simulink model "fuzzy_TCLAB_toolbox"  (R2021a)
settings: Solver=ode45  StartTime=0.0  StopTime=600  RelTol=1e-3  EnableMultiTasking=on
libraries: fuzblock x1
settings Model: Creator=Sergio  LastModifiedBy=Sergio
settings SolverCC: AlgebraicLoopSolver=TrustRegion
settings DataIOCC: LimitDataPoints=on  SaveFormat=Array  SignalLoggingSaveFormat=ModelDataLogs  ReturnWorkspaceOutputs=off
settings OptimizationCC: ExpressionDepthLimit=2147483647  LifeSpan=inf
settings DebuggingCC: UnderspecifiedInitializationDetection=Classic  MergeDetectMultiDrivingBlocksExec=none  SolverPrmCheckMsg=warning  FcnCallInpInsideContextMsg=warning  StateNameClashWarn=warning  SFUnexpectedBacktrackingDiag=warning  SFNoUnconditionalDefaultTransitionDiag=warning  SFExecutionAtInitializationDiag=none  SFMachineParentedDataDiag=warning  ArithmeticOperatorsInVariantConditions=warning
settings HardwareCC: ProdBitPerPointer=32  ProdBitPerSizeT=32  ProdBitPerPtrDiffT=32  ProdLargestAtomicFloat=None  ProdIntDivRoundTo=Undefined  ProdEndianess=Unspecified  ProdWordSize=32  ProdHWDeviceType=32-bit Generic
settings ModelReferenceCC: PropagateSignalLabelsOutOfModel=off
settings SFSimCC: SimUseLocalCustomCode=off  CustomCodeUndefinedFunction=UseInterfaceOnly
settings RTWCC: RTWUseLocalCustomCode=off
settings CodeAppCC: StateflowObjectComments=on
settings GRTTargetCC: TargetLangStandard=C89/C90 (ANSI)  CombineOutputUpdateFcns=off  GRTInterface=on
settings ConfigComp: CovMetricSettings=dw  CovSaveCumulativeToWorkspaceVar=on  CovSaveSingleToWorkspaceVar=on  CovExternalEMLEnable=off

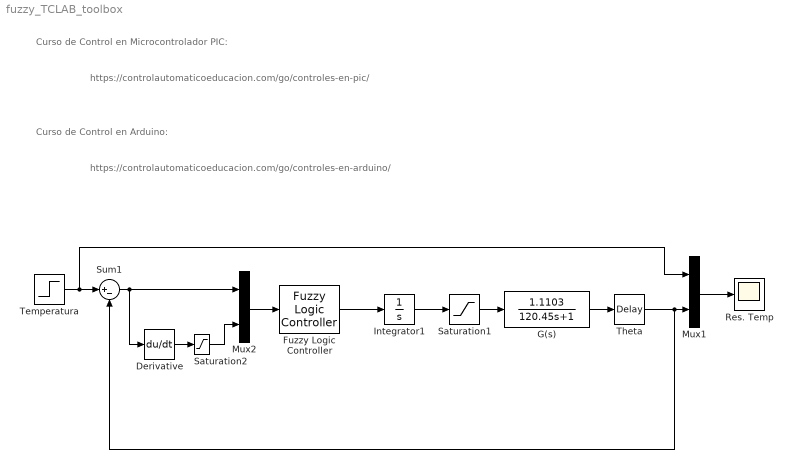
== system fuzzy_TCLAB_toolbox ==
  note: https://controlautomaticoeducacion.com/go/controles-en-pic/
  note: Curso de Control en Microcontrolador PIC:
  note: https://controlautomaticoeducacion.com/go/controles-en-arduino/
  note: Curso de Control en Arduino:
  Derivative : Derivative
  Fuzzy Logic Controller : fuzblock/Fuzzy Logic  Controller  FIS=PI_FUZZY  OutputSampleNumber=101  DataType=double  FuzzifiedInputs=off  RuleFiringStrengths=off  RuleOutputs=off  AggregatedOutputs=off  SimulateUsing=Interpreted execution  OutOfRangeInputValueMessage=warning  NoRuleFiredMessage=warning  EmptyOutputFuzzySetMessage=warning
  G(s) : TransferFcn  Numerator=[1.1103]  Denominator=[120.45 1]
  Integrator1 : Integrator
  Mux1 : Mux  Inputs=2
  Mux2 : Mux  Inputs=2
  Res. Temp : Scope
  Saturation1 : Saturate  UpperLimit=100  LowerLimit=0
  Saturation2 : Saturate  UpperLimit=4  LowerLimit=-4
  Sum1 : Sum  Inputs=|+-
  Temperatura : Step  Time=0  After=50  SampleTime=0
  Theta : TransportDelay  DelayTime=12.78
  wires:
  Temperatura/1 -> Sum1/1, Mux1/1
  G(s)/1 -> Theta/1
  Theta/1 -> Mux1/2, Sum1/2
  Mux1/1 -> Res. Temp/1
  Mux2/1 -> Fuzzy Logic Controller/1
  Sum1/1 -> Mux2/1, Derivative/1
  Fuzzy Logic Controller/1 -> Integrator1/1
  Integrator1/1 -> Saturation1/1
  Saturation1/1 -> G(s)/1
  Saturation2/1 -> Mux2/2
  Derivative/1 -> Saturation2/1
